simulink model "grid"  (R2014b)
settings: Solver=ode45  StartTime=0.0  StopTime=0.5  RelTol=1e-3
undefined symbols (not defined in the file): D1, Delta
libraries: powerlib x104, simulink x30
(part 1 of 2)
settings Model: Creator=quad  LastModifiedBy=SELVA
settings DataIOCC: SignalLoggingSaveFormat=ModelDataLogs
settings OptimizationCC: ExpressionDepthLimit=2147483647
settings DebuggingCC: UnderspecifiedInitializationDetection=Classic  MergeDetectMultiDrivingBlocksExec=none  FcnCallInpInsideContextMsg=UseLocalSettings  StateNameClashWarn=warning
settings GRTTargetCC: CombineOutputUpdateFcns=off  GRTInterface=on

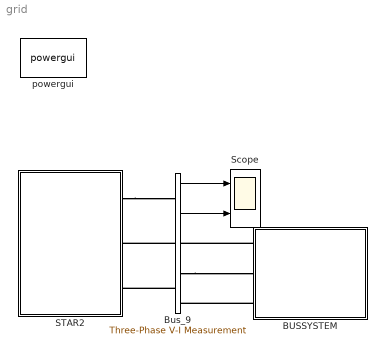
== system grid ==
  BUSSYSTEM : Subsystem
  Bus_9 : powerlib/Measurements/Three-Phase V-I Measurement  VoltageMeasurement=phase-to-phase  SetLabelV=off  LabelV=Vabc_12  Vpu=off  VpuLL=off  CurrentMeasurement=yes  SetLabelI=off  LabelI=Iabc_12  Ipu=off  Pbase=100e6  Vbase=120e3  OutputType=Complex  PhasorSimulation=on  PSBequivalent=0
  STAR2 : Subsystem
  Scope : Scope  NumInputPorts=2
      settings: YMin=-800~-3000  YMax=800~3000
  powergui : powerlib/powergui  Priority=1  SimulationMode=Discrete  SolverType=Tustin/Backward Euler (TBE)  SampleTime=5e-6  frequency=60  SPID=off  DisableSnubberDevices=off  DisableRonSwitches=off  DisableVfSwitches=off  SwTol=0  DisplayEquations=off  Interpol=off  methode=off  Ts=100  frequencyindice=50  Pbase=100e6  ErrMax=1e-4  Iterations=50  UnitsV=kV  UnitsW=MW  FunctionMessages=off  echomessages=off  HookPort=off  EnableUseOfTLC=off  x0status=blocks  RestoreLinks=warning  ResistiveCurrentMeasurement=off  Frange=[0:2:500]  Ylog=off  Xlog=on  ShowGrid=off  save=off  variable=ZData  structure=bn  ZoomFFT=off  StartTime=0.0  cycles=1  DisplayStyle=1  fundamental=60  FreqAxis=off  MaxFrequency=1000  frequencyindicesteady=1  RmsSteady=1  display=off
  wires:
  Bus_9/2 -> Scope/2
  Bus_9/1 -> Scope/1
  connections:
  STAR2/RConn1 -- Bus_9/LConn1
  Bus_9/LConn2 -- STAR2/RConn2
  Bus_9/LConn3 -- STAR2/RConn3
  BUSSYSTEM/LConn1 -- Bus_9/RConn1
  Bus_9/RConn2 -- BUSSYSTEM/LConn2
  BUSSYSTEM/LConn3 -- Bus_9/RConn3

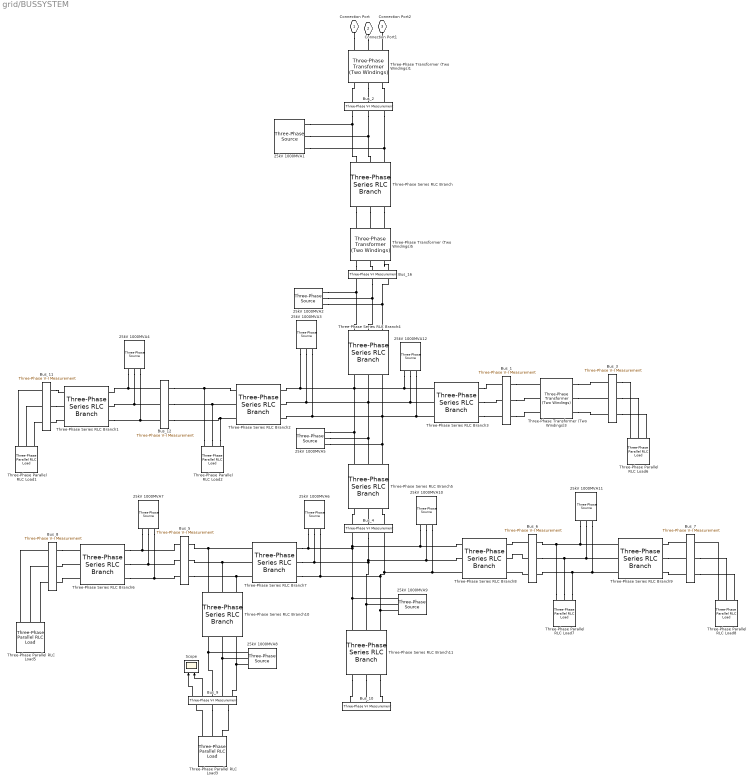
== system grid/BUSSYSTEM ==
  25kV 1000MVA{1..4,6..12} (11 alike) : powerlib/Electrical Sources/Three-Phase Source  Voltage=10  PhaseAngle=0  Frequency=50  InternalConnection=Yg  SpecifyImpedance=on  Resistance=25^2/1000/10  Inductance=25^2/1000/377  ShortCircuitLevel=1000e6  BaseVoltage=25e3  XRratio=10  BusType=swing  Pref=0  Qref=0  Qmin=-inf  Qmax=inf
  25kV 1000MVA5 : powerlib/Electrical Sources/Three-Phase Source  Voltage=25e3  PhaseAngle=0  Frequency=50  InternalConnection=Yg  SpecifyImpedance=on  Resistance=25^2/1000/10  Inductance=25^2/1000/377  ShortCircuitLevel=1000e6  BaseVoltage=25e3  XRratio=10  BusType=swing  Pref=0  Qref=0  Qmin=-inf  Qmax=inf
  Bus_1 : powerlib/Measurements/Three-Phase V-I Measurement  VoltageMeasurement=phase-to-phase  SetLabelV=on  LabelV=Vabc_5  Vpu=off  VpuLL=off  CurrentMeasurement=yes  SetLabelI=on  LabelI=Iabc_5  Ipu=off  Pbase=100e6  Vbase=120e3  OutputType=Complex  PhasorSimulation=on  PSBequivalent=0
  Bus_10 : powerlib/Measurements/Three-Phase V-I Measurement  VoltageMeasurement=phase-to-phase  SetLabelV=on  LabelV=Vabc_13  Vpu=off  VpuLL=off  CurrentMeasurement=yes  SetLabelI=on  LabelI=Iabc_13  Ipu=off  Pbase=100e6  Vbase=120e3  OutputType=Complex  PhasorSimulation=on  PSBequivalent=0
  Bus_11 : powerlib/Measurements/Three-Phase V-I Measurement  VoltageMeasurement=phase-to-phase  SetLabelV=on  LabelV=Vabc_3  Vpu=off  VpuLL=off  CurrentMeasurement=yes  SetLabelI=on  LabelI=Iabc_3  Ipu=off  Pbase=100e6  Vbase=120e3  OutputType=Complex  PhasorSimulation=on  PSBequivalent=0
  Bus_12 : powerlib/Measurements/Three-Phase V-I Measurement  VoltageMeasurement=phase-to-phase  SetLabelV=on  LabelV=Vabc_4  Vpu=off  VpuLL=off  CurrentMeasurement=yes  SetLabelI=on  LabelI=Iabc_4  Ipu=off  Pbase=100e6  Vbase=120e3  OutputType=Complex  PhasorSimulation=on  PSBequivalent=0
  Bus_16 : powerlib/Measurements/Three-Phase V-I Measurement  VoltageMeasurement=phase-to-phase  SetLabelV=on  LabelV=Vabc_1  Vpu=off  VpuLL=off  CurrentMeasurement=yes  SetLabelI=on  LabelI=Iabc_1  Ipu=off  Pbase=100e6  Vbase=120e3  OutputType=Complex  PhasorSimulation=on  PSBequivalent=0
  Bus_2 : powerlib/Measurements/Three-Phase V-I Measurement  VoltageMeasurement=phase-to-phase  SetLabelV=on  LabelV=Vabc_2  Vpu=off  VpuLL=off  CurrentMeasurement=yes  SetLabelI=on  LabelI=Iabc_2  Ipu=off  Pbase=100e6  Vbase=120e3  OutputType=Complex  PhasorSimulation=on  PSBequivalent=0
  Bus_3 : powerlib/Measurements/Three-Phase V-I Measurement  VoltageMeasurement=phase-to-phase  SetLabelV=on  LabelV=Vabc_6  Vpu=off  VpuLL=off  CurrentMeasurement=yes  SetLabelI=on  LabelI=Iabc_6  Ipu=off  Pbase=100e6  Vbase=120e3  OutputType=Complex  PhasorSimulation=on  PSBequivalent=0
  Bus_4 : powerlib/Measurements/Three-Phase V-I Measurement  VoltageMeasurement=phase-to-phase  SetLabelV=on  LabelV=Vabc_7  Vpu=off  VpuLL=off  CurrentMeasurement=yes  SetLabelI=on  LabelI=Iabc_7  Ipu=off  Pbase=100e6  Vbase=120e3  OutputType=Complex  PhasorSimulation=on  PSBequivalent=0
  Bus_5 : powerlib/Measurements/Three-Phase V-I Measurement  VoltageMeasurement=phase-to-phase  SetLabelV=on  LabelV=Vabc_8  Vpu=off  VpuLL=off  CurrentMeasurement=yes  SetLabelI=on  LabelI=Iabc_8  Ipu=off  Pbase=100e6  Vbase=120e3  OutputType=Complex  PhasorSimulation=on  PSBequivalent=0
  Bus_6 : powerlib/Measurements/Three-Phase V-I Measurement  VoltageMeasurement=phase-to-phase  SetLabelV=on  LabelV=Vabc_10  Vpu=off  VpuLL=off  CurrentMeasurement=yes  SetLabelI=on  LabelI=Iabc_10  Ipu=off  Pbase=100e6  Vbase=120e3  OutputType=Complex  PhasorSimulation=on  PSBequivalent=0
  Bus_7 : powerlib/Measurements/Three-Phase V-I Measurement  VoltageMeasurement=phase-to-phase  SetLabelV=on  LabelV=Vabc_11  Vpu=off  VpuLL=off  CurrentMeasurement=yes  SetLabelI=on  LabelI=Iabc_11  Ipu=off  Pbase=100e6  Vbase=120e3  OutputType=Complex  PhasorSimulation=on  PSBequivalent=0
  Bus_8 : powerlib/Measurements/Three-Phase V-I Measurement  VoltageMeasurement=phase-to-phase  SetLabelV=on  LabelV=Vabc_9  Vpu=off  VpuLL=off  CurrentMeasurement=yes  SetLabelI=on  LabelI=Iabc_9  Ipu=off  Pbase=100e6  Vbase=120e3  OutputType=Complex  PhasorSimulation=on  PSBequivalent=0
  Bus_9 : powerlib/Measurements/Three-Phase V-I Measurement  VoltageMeasurement=phase-to-phase  SetLabelV=off  LabelV=Vabc_12  Vpu=off  VpuLL=off  CurrentMeasurement=yes  SetLabelI=off  LabelI=Iabc_12  Ipu=off  Pbase=100e6  Vbase=120e3  OutputType=Complex  PhasorSimulation=on  PSBequivalent=0
  Scope : Scope  NumInputPorts=2
      settings: YMin=-15~-0.5  YMax=15~0.5  SaveName=ScopeData4
  Three-Phase Parallel RLC Load{1..3,5..8} (7 alike) : powerlib/Elements/Three-Phase Parallel RLC Load  LConnTagsString=A|B|C  Configuration=Y (grounded)  NominalVoltage=415  NominalFrequency=50  ActivePower=10e3  InductivePower=0  CapacitivePower=0  Measurements=None  LoadType=constant Z
  Three-Phase Series RLC Branch{,1..11} (12 alike) : powerlib/Elements/Three-Phase Series RLC Branch  LConnTagsString=A|B|C  RConnTagsString=A|B|C  BranchType=RL  Resistance=10  Inductance=1e-3  Capacitance=1e-6  Measurements=None
  Three-Phase Transformer (Two Windings)1 : powerlib/Elements/Three-Phase Transformer (Two Windings)  Winding1Connection=Delta (D1)  UNITS=pu  NominalPower=[ 1 , 50 ]  Winding1=[1.06 0.002 0.08]  Winding2Connection=Yg  Winding2=[100 0.002 0.080001]  SetSaturation=off  Rm=500  Lm=500  Saturation=[0 0;0.0023999 1.2;1 1.52]  Hysteresis=off  DataFile='hysteresis'  SetInitialFlux=off  InitialFluxes=[0.79999 -0.79999 0.70001]  Measurements=None  MoreParameters=off  BreakLoop=off  DataType=off  TransfoNumber=1
  Three-Phase Transformer (Two Windings)3 : powerlib/Elements/Three-Phase Transformer (Two Windings)  Winding1Connection=Delta (D1)  UNITS=pu  NominalPower=[ 1 , 50 ]  Winding1=[ 1.06 , 0.002 , 0.08 ]  Winding2Connection=Yg  Winding2=[ 1.06 , 0.002 , 0.08 ]  SetSaturation=off  Rm=500  Lm=500  Saturation=[ 0,0 ; 0.0024,1.2 ; 1.0,1.52 ]  Hysteresis=off  DataFile='hysteresis'  SetInitialFlux=off  InitialFluxes=[ 0.8 , -0.8 , 0.7 ]  Measurements=None  MoreParameters=off  BreakLoop=off  DataType=off  TransfoNumber=1
  Three-Phase Transformer (Two Windings)5 : powerlib/Elements/Three-Phase Transformer (Two Windings)  Winding1Connection=Delta (D1)  UNITS=pu  NominalPower=[ 1 , 50 ]  Winding1=[ 1.06 , 0.002 , 0.08 ]  Winding2Connection=Yg  Winding2=[1000 , 0.002 , 0.08 ]  SetSaturation=off  Rm=500  Lm=500  Saturation=[ 0,0 ; 0.0024,1.2 ; 1.0,1.52 ]  Hysteresis=off  DataFile='hysteresis'  SetInitialFlux=off  InitialFluxes=[ 0.8 , -0.8 , 0.7 ]  Measurements=None  MoreParameters=off  BreakLoop=off  DataType=off  TransfoNumber=1
  Connection Port : PMIOPort  Tag=PMCPort  Port=1  Side=Left
  Connection Port1 : PMIOPort  Tag=PMCPort  Port=2  Side=Left
  Connection Port2 : PMIOPort  Tag=PMCPort  Port=3  Side=Left
  wires:
  Bus_9/1 -> Scope/1
  Bus_9/2 -> Scope/2
  connections:
  Three-Phase Parallel RLC Load2/LConn3 -- Bus_12/RConn3 -- Three-Phase Series RLC Branch2/LConn3
  Three-Phase Parallel RLC Load2/LConn2 -- Three-Phase Series RLC Branch2/LConn2 -- Bus_12/RConn2
  Three-Phase Parallel RLC Load2/LConn1 -- Bus_12/RConn1 -- Three-Phase Series RLC Branch2/LConn1
  Three-Phase Series RLC Branch10/RConn2 -- Bus_5/RConn2 -- Three-Phase Series RLC Branch7/LConn2
  Three-Phase Series RLC Branch10/RConn3 -- Bus_5/RConn3 -- Three-Phase Series RLC Branch7/LConn3
  Three-Phase Series RLC Branch10/RConn1 -- Bus_5/RConn1 -- Three-Phase Series RLC Branch7/LConn1
  25kV 1000MVA12/RConn1 -- Three-Phase Series RLC Branch4/RConn1 -- Three-Phase Series RLC Branch2/RConn1 -- 25kV 1000MVA3/RConn1 -- Three-Phase Series RLC Branch5/LConn1 -- 25kV 1000MVA5/RConn1 -- Three-Phase Series RLC Branch3/LConn1
  25kV 1000MVA12/RConn2 -- Three-Phase Series RLC Branch2/RConn2 -- 25kV 1000MVA3/RConn2 -- Three-Phase Series RLC Branch4/RConn2 -- Three-Phase Series RLC Branch5/LConn2 -- 25kV 1000MVA5/RConn2 -- Three-Phase Series RLC Branch3/LConn2
  25kV 1000MVA12/RConn3 -- Three-Phase Series RLC Branch4/RConn3 -- Three-Phase Series RLC Branch2/RConn3 -- 25kV 1000MVA3/RConn3 -- Three-Phase Series RLC Branch5/LConn3 -- 25kV 1000MVA5/RConn3 -- Three-Phase Series RLC Branch3/LConn3
  25kV 1000MVA10/RConn1 -- Three-Phase Series RLC Branch7/RConn1 -- 25kV 1000MVA6/RConn1 -- Three-Phase Series RLC Branch11/LConn1 -- 25kV 1000MVA9/RConn1 -- Bus_4/LConn1 -- Three-Phase Series RLC Branch8/LConn1
  25kV 1000MVA10/RConn2 -- Three-Phase Series RLC Branch7/RConn2 -- 25kV 1000MVA6/RConn2 -- Three-Phase Series RLC Branch11/LConn2 -- 25kV 1000MVA9/RConn2 -- Bus_4/LConn2 -- Three-Phase Series RLC Branch8/LConn2
  25kV 1000MVA10/RConn3 -- Bus_4/LConn3 -- Three-Phase Series RLC Branch7/RConn3 -- 25kV 1000MVA6/RConn3 -- Three-Phase Series RLC Branch11/LConn3 -- 25kV 1000MVA9/RConn3 -- Three-Phase Series RLC Branch8/LConn3
  25kV 1000MVA4/RConn3 -- Three-Phase Series RLC Branch1/RConn3 -- Bus_12/LConn3
  25kV 1000MVA1/RConn3 -- Bus_2/LConn3 -- Three-Phase Series RLC Branch/LConn3
  25kV 1000MVA8/RConn3 -- Bus_9/RConn3 -- Three-Phase Series RLC Branch10/LConn3
  Three-Phase Parallel RLC Load7/LConn1 -- Bus_6/RConn1 -- Three-Phase Series RLC Branch9/LConn1 -- 25kV 1000MVA11/RConn1
  25kV 1000MVA4/RConn1 -- Three-Phase Series RLC Branch1/RConn1 -- Bus_12/LConn1
  25kV 1000MVA2/RConn2 -- Bus_16/LConn2 -- Three-Phase Series RLC Branch4/LConn2
  25kV 1000MVA2/RConn3 -- Bus_16/LConn3 -- Three-Phase Series RLC Branch4/LConn3
  25kV 1000MVA8/RConn1 -- Bus_9/RConn1 -- Three-Phase Series RLC Branch10/LConn1
  25kV 1000MVA2/RConn1 -- Bus_16/LConn1 -- Three-Phase Series RLC Branch4/LConn1
  25kV 1000MVA4/RConn2 -- Three-Phase Series RLC Branch1/RConn2 -- Bus_12/LConn2
  25kV 1000MVA7/RConn1 -- Three-Phase Series RLC Branch6/RConn1 -- Bus_5/LConn1
  Three-Phase Parallel RLC Load7/LConn2 -- Bus_6/RConn2 -- Three-Phase Series RLC Branch9/LConn2 -- 25kV 1000MVA11/RConn2
  25kV 1000MVA8/RConn2 -- Bus_9/RConn2 -- Three-Phase Series RLC Branch10/LConn2
  25kV 1000MVA1/RConn2 -- Bus_2/LConn2 -- Three-Phase Series RLC Branch/LConn2
  25kV 1000MVA1/RConn1 -- Bus_2/LConn1 -- Three-Phase Series RLC Branch/LConn1
  25kV 1000MVA7/RConn2 -- Three-Phase Series RLC Branch6/RConn2 -- Bus_5/LConn2
  25kV 1000MVA7/RConn3 -- Three-Phase Series RLC Branch6/RConn3 -- Bus_5/LConn3
  Three-Phase Parallel RLC Load7/LConn3 -- Bus_6/RConn3 -- Three-Phase Series RLC Branch9/LConn3 -- 25kV 1000MVA11/RConn3
  Three-Phase Series RLC Branch/RConn1 -- Three-Phase Transformer (Two Windings)5/LConn1
  Bus_7/RConn2 -- Three-Phase Parallel RLC Load8/LConn2
  Three-Phase Parallel RLC Load1/LConn2 -- Bus_11/LConn2
  Three-Phase Series RLC Branch5/RConn3 -- Bus_4/RConn3
  Three-Phase Transformer (Two Windings)3/LConn3 -- Bus_3/LConn3
  Bus_6/LConn2 -- Three-Phase Series RLC Branch8/RConn2
  Bus_1/RConn2 -- Three-Phase Transformer (Two Windings)3/RConn2
  Bus_11/RConn3 -- Three-Phase Series RLC Branch1/LConn3
  Bus_6/LConn3 -- Three-Phase Series RLC Branch8/RConn3
  Bus_8/RConn2 -- Three-Phase Series RLC Branch6/LConn2
  Three-Phase Parallel RLC Load5/LConn2 -- Bus_8/LConn2
  Three-Phase Series RLC Branch/RConn3 -- Three-Phase Transformer (Two Windings)5/LConn3
  Bus_7/RConn3 -- Three-Phase Parallel RLC Load8/LConn3
  Bus_3/RConn1 -- Three-Phase Parallel RLC Load6/LConn1
  Three-Phase Parallel RLC Load8/LConn1 -- Bus_7/RConn1
  Three-Phase Parallel RLC Load5/LConn1 -- Bus_8/LConn1
  Three-Phase Series RLC Branch11/RConn1 -- Bus_10/RConn1
  Three-Phase Transformer (Two Windings)1/RConn3 -- Bus_2/RConn3
  Three-Phase Series RLC Branch9/RConn2 -- Bus_7/LConn2
  Bus_11/RConn2 -- Three-Phase Series RLC Branch1/LConn2
  Three-Phase Series RLC Branch3/RConn3 -- Bus_1/LConn3
  Bus_9/LConn2 -- Three-Phase Parallel RLC Load3/LConn2
  Three-Phase Transformer (Two Windings)3/LConn1 -- Bus_3/LConn1
  Three-Phase Series RLC Branch3/RConn1 -- Bus_1/LConn1
  Three-Phase Parallel RLC Load5/LConn3 -- Bus_8/LConn3
  Three-Phase Parallel RLC Load1/LConn3 -- Bus_11/LConn3
  Three-Phase Transformer (Two Windings)5/RConn2 -- Bus_16/RConn2
  Three-Phase Series RLC Branch3/RConn2 -- Bus_1/LConn2
  Three-Phase Series RLC Branch9/RConn3 -- Bus_7/LConn3
  Bus_9/LConn3 -- Three-Phase Parallel RLC Load3/LConn3
  Bus_6/LConn1 -- Three-Phase Series RLC Branch8/RConn1
  Bus_1/RConn3 -- Three-Phase Transformer (Two Windings)3/RConn3
  Bus_4/RConn2 -- Three-Phase Series RLC Branch5/RConn2
  Bus_3/RConn3 -- Three-Phase Parallel RLC Load6/LConn3
  Bus_8/RConn3 -- Three-Phase Series RLC Branch6/LConn3
  Three-Phase Series RLC Branch11/RConn2 -- Bus_10/RConn2
  Bus_1/RConn1 -- Three-Phase Transformer (Two Windings)3/RConn1
  Three-Phase Series RLC Branch11/RConn3 -- Bus_10/RConn3
  Three-Phase Transformer (Two Windings)3/LConn2 -- Bus_3/LConn2
  Three-Phase Transformer (Two Windings)1/RConn2 -- Bus_2/RConn2
  Bus_3/RConn2 -- Three-Phase Parallel RLC Load6/LConn2
  Three-Phase Transformer (Two Windings)5/RConn1 -- Bus_16/RConn1
  Three-Phase Series RLC Branch9/RConn1 -- Bus_7/LConn1
  Three-Phase Parallel RLC Load3/LConn1 -- Bus_9/LConn1
  Bus_11/RConn1 -- Three-Phase Series RLC Branch1/LConn1
  Three-Phase Parallel RLC Load1/LConn1 -- Bus_11/LConn1
  Bus_4/RConn1 -- Three-Phase Series RLC Branch5/RConn1
  Three-Phase Transformer (Two Windings)1/RConn1 -- Bus_2/RConn1
  Three-Phase Series RLC Branch/RConn2 -- Three-Phase Transformer (Two Windings)5/LConn2
  Three-Phase Transformer (Two Windings)5/RConn3 -- Bus_16/RConn3
  Connection Port1/RConn1 -- Three-Phase Transformer (Two Windings)1/LConn2
  Bus_8/RConn1 -- Three-Phase Series RLC Branch6/LConn1
  Connection Port/RConn1 -- Three-Phase Transformer (Two Windings)1/LConn1
  Connection Port2/RConn1 -- Three-Phase Transformer (Two Windings)1/LConn3

== system grid/STAR2 ==
  "B " : Subsystem
  DC : Subsystem
  DC1 : Subsystem
  DC2 : Subsystem
  Ground : powerlib/Elements/Ground  LConnTagsString=a
  R : Subsystem
  Y : Subsystem
  A : PMIOPort  Tag=PMCPort  Port=1  Side=Right
  B : PMIOPort  Tag=PMCPort  Port=2  Side=Right
  C : PMIOPort  Tag=PMCPort  Port=3  Side=Right
  connections:
  R/RConn2 -- Y/RConn2 -- "B "/RConn2 -- Ground/LConn1
  DC/RConn1 -- R/LConn1
  DC/RConn3 -- R/LConn3
  DC/RConn4 -- R/LConn4
  DC/RConn9 -- R/LConn9
  DC/RConn2 -- R/LConn2
  DC/RConn5 -- R/LConn5
  DC/RConn7 -- R/LConn7
  DC/RConn6 -- R/LConn6
  DC/RConn8 -- R/LConn8
  DC/RConn10 -- R/LConn10
  DC1/RConn1 -- Y/LConn1
  DC1/RConn2 -- Y/LConn2
  DC1/RConn3 -- Y/LConn3
  DC1/RConn4 -- Y/LConn4
  DC1/RConn5 -- Y/LConn5
  DC1/RConn6 -- Y/LConn6
  DC1/RConn7 -- Y/LConn7
  DC1/RConn8 -- Y/LConn8
  DC1/RConn9 -- Y/LConn9
  DC1/RConn10 -- Y/LConn10
  DC2/RConn1 -- "B "/LConn1
  DC2/RConn2 -- "B "/LConn2
  DC2/RConn3 -- "B "/LConn3
  DC2/RConn4 -- "B "/LConn4
  DC2/RConn5 -- "B "/LConn5
  DC2/RConn6 -- "B "/LConn6
  DC2/RConn7 -- "B "/LConn7
  DC2/RConn8 -- "B "/LConn8
  DC2/RConn9 -- "B "/LConn9
  DC2/RConn10 -- "B "/LConn10
  Y/RConn1 -- B/RConn1
  R/RConn1 -- A/RConn1
  "B "/RConn1 -- C/RConn1

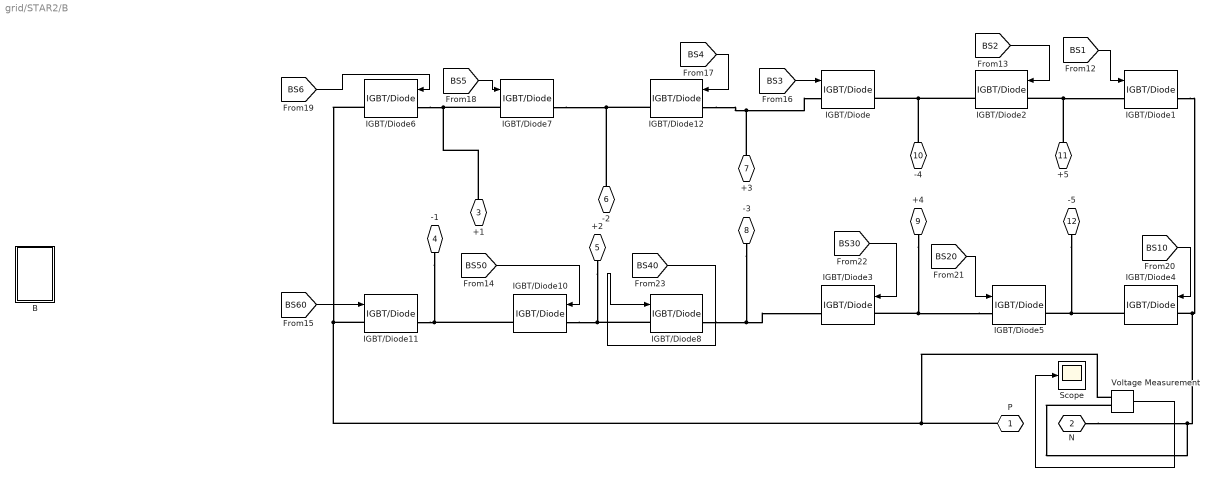
== system grid/STAR2/B  ==
  B : Subsystem  mask{fc=1000, m=1}
      mask prompts: fc "Switching frequency"; m "modulation index"
  IGBT/Diode{,1..8,10..12} (12 alike) : powerlib/Power Electronics/IGBT//Diode  Ron=1e-3  Rs=1e5  Cs=inf  Measurements=on
  Scope : Scope
  Voltage Measurement : powerlib/Measurements/Voltage Measurement  PhasorSimulation=off  OutputType=Complex  PSBequivalent=0
  P : PMIOPort  Tag=PMCPort  Port=1  Side=Right
  N : PMIOPort  Tag=PMCPort  Port=2  Side=Right
  +1 : PMIOPort  Tag=PMCPort  Port=3  Side=Left
  -1 : PMIOPort  Tag=PMCPort  Port=4  Side=Left
  +2 : PMIOPort  Tag=PMCPort  Port=5  Side=Left
  -2 : PMIOPort  Tag=PMCPort  Port=6  Side=Left
  +3 : PMIOPort  Tag=PMCPort  Port=7  Side=Left
  -3 : PMIOPort  Tag=PMCPort  Port=8  Side=Left
  +4 : PMIOPort  Tag=PMCPort  Port=9  Side=Left
  -4 : PMIOPort  Tag=PMCPort  Port=10  Side=Left
  +5 : PMIOPort  Tag=PMCPort  Port=11  Side=Left
  -5 : PMIOPort  Tag=PMCPort  Port=12  Side=Left
  wires:
  [BS10] -> IGBT/Diode4/1
  [BS2] -> IGBT/Diode2/1
  [BS20] -> IGBT/Diode5/1
  [BS3] -> IGBT/Diode/1
  [BS30] -> IGBT/Diode3/1
  [BS40] -> IGBT/Diode8/1
  [BS6] -> IGBT/Diode6/1
  [BS4] -> IGBT/Diode12/1
  [BS5] -> IGBT/Diode7/1
  [BS50] -> IGBT/Diode10/1
  [BS60] -> IGBT/Diode11/1
  Voltage Measurement/1 -> Scope/1
  [BS1] -> IGBT/Diode1/1
  connections:
  IGBT/Diode2/RConn1 -- -4/RConn1 -- IGBT/Diode/RConn1
  IGBT/Diode2/LConn1 -- IGBT/Diode1/LConn1 -- +5/RConn1
  IGBT/Diode5/LConn1 -- +4/RConn1 -- IGBT/Diode3/LConn1
  IGBT/Diode4/RConn1 -- -5/RConn1 -- IGBT/Diode5/RConn1
  IGBT/Diode4/LConn1 -- IGBT/Diode1/RConn1 -- N/RConn1 -- Voltage Measurement/LConn2
  IGBT/Diode7/LConn1 -- +1/RConn1 -- IGBT/Diode6/LConn1
  IGBT/Diode12/RConn1 -- IGBT/Diode7/RConn1 -- -2/RConn1
  IGBT/Diode10/RConn1 -- IGBT/Diode11/RConn1 -- -1/RConn1
  IGBT/Diode8/LConn1 -- IGBT/Diode10/LConn1 -- +2/RConn1
  IGBT/Diode12/LConn1 -- IGBT/Diode/LConn1 -- +3/RConn1
  IGBT/Diode8/RConn1 -- IGBT/Diode3/RConn1 -- -3/RConn1
  IGBT/Diode6/RConn1 -- IGBT/Diode11/LConn1 -- P/RConn1 -- Voltage Measurement/LConn1

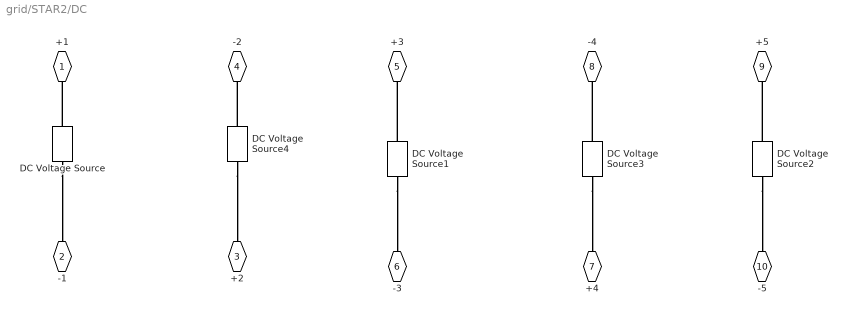
== system grid/STAR2/DC ==
  DC Voltage Source{,1..4} (5 alike) : powerlib/Electrical Sources/DC Voltage Source  Amplitude=66.5  Measurements=None
  +1 : PMIOPort  Tag=PMCPort  Port=1  Side=Right
  -1 : PMIOPort  Tag=PMCPort  Port=2  Side=Right
  +2 : PMIOPort  Tag=PMCPort  Port=3  Side=Right
  -2 : PMIOPort  Tag=PMCPort  Port=4  Side=Right
  +3 : PMIOPort  Tag=PMCPort  Port=5  Side=Right
  -3 : PMIOPort  Tag=PMCPort  Port=6  Side=Right
  +4 : PMIOPort  Tag=PMCPort  Port=7  Side=Right
  -4 : PMIOPort  Tag=PMCPort  Port=8  Side=Right
  +5 : PMIOPort  Tag=PMCPort  Port=9  Side=Right
  -5 : PMIOPort  Tag=PMCPort  Port=10  Side=Right
  connections:
  DC Voltage Source/LConn1 -- -1/RConn1
  DC Voltage Source/RConn1 -- +1/RConn1
  DC Voltage Source1/LConn1 -- -3/RConn1
  DC Voltage Source3/RConn1 -- +4/RConn1
  DC Voltage Source2/LConn1 -- -5/RConn1
  DC Voltage Source1/RConn1 -- +3/RConn1
  DC Voltage Source2/RConn1 -- +5/RConn1
  DC Voltage Source3/LConn1 -- -4/RConn1
  DC Voltage Source4/LConn1 -- -2/RConn1
  DC Voltage Source4/RConn1 -- +2/RConn1

== system grid/STAR2/DC1 ==
  DC Voltage Source{,1..4} (5 alike) : powerlib/Electrical Sources/DC Voltage Source  Amplitude=66.5  Measurements=None
  +1 : PMIOPort  Tag=PMCPort  Port=1  Side=Right
  -1 : PMIOPort  Tag=PMCPort  Port=2  Side=Right
  +2 : PMIOPort  Tag=PMCPort  Port=3  Side=Right
  -2 : PMIOPort  Tag=PMCPort  Port=4  Side=Right
  +3 : PMIOPort  Tag=PMCPort  Port=5  Side=Right
  -3 : PMIOPort  Tag=PMCPort  Port=6  Side=Right
  +4 : PMIOPort  Tag=PMCPort  Port=7  Side=Right
  -4 : PMIOPort  Tag=PMCPort  Port=8  Side=Right
  +5 : PMIOPort  Tag=PMCPort  Port=9  Side=Right
  -5 : PMIOPort  Tag=PMCPort  Port=10  Side=Right
  connections:
  DC Voltage Source4/RConn1 -- +2/RConn1
  DC Voltage Source4/LConn1 -- -2/RConn1
  DC Voltage Source3/LConn1 -- -4/RConn1
  DC Voltage Source2/RConn1 -- +5/RConn1
  DC Voltage Source1/RConn1 -- +3/RConn1
  DC Voltage Source2/LConn1 -- -5/RConn1
  DC Voltage Source3/RConn1 -- +4/RConn1
  DC Voltage Source1/LConn1 -- -3/RConn1
  DC Voltage Source/RConn1 -- +1/RConn1
  DC Voltage Source/LConn1 -- -1/RConn1

== system grid/STAR2/DC2 ==
  DC Voltage Source{,1..4} (5 alike) : powerlib/Electrical Sources/DC Voltage Source  Amplitude=66.5  Measurements=None
  +1 : PMIOPort  Tag=PMCPort  Port=1  Side=Right
  -1 : PMIOPort  Tag=PMCPort  Port=2  Side=Right
  +2 : PMIOPort  Tag=PMCPort  Port=3  Side=Right
  -2 : PMIOPort  Tag=PMCPort  Port=4  Side=Right
  +3 : PMIOPort  Tag=PMCPort  Port=5  Side=Right
  -3 : PMIOPort  Tag=PMCPort  Port=6  Side=Right
  +4 : PMIOPort  Tag=PMCPort  Port=7  Side=Right
  -4 : PMIOPort  Tag=PMCPort  Port=8  Side=Right
  +5 : PMIOPort  Tag=PMCPort  Port=9  Side=Right
  -5 : PMIOPort  Tag=PMCPort  Port=10  Side=Right
  connections:
  DC Voltage Source/LConn1 -- -1/RConn1
  DC Voltage Source/RConn1 -- +1/RConn1
  DC Voltage Source1/LConn1 -- -3/RConn1
  DC Voltage Source3/RConn1 -- +4/RConn1
  DC Voltage Source2/LConn1 -- -5/RConn1
  DC Voltage Source1/RConn1 -- +3/RConn1
  DC Voltage Source2/RConn1 -- +5/RConn1
  DC Voltage Source3/LConn1 -- -4/RConn1
  DC Voltage Source4/LConn1 -- -2/RConn1
  DC Voltage Source4/RConn1 -- +2/RConn1

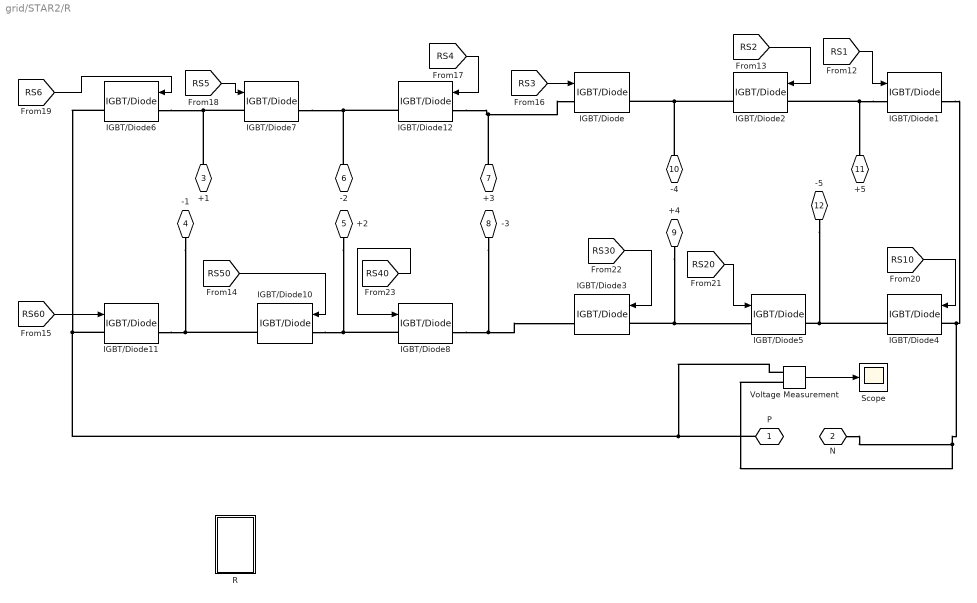
== system grid/STAR2/R ==
  IGBT/Diode{,1..8,10..12} (12 alike) : powerlib/Power Electronics/IGBT//Diode  Ron=1e-3  Rs=1e5  Cs=inf  Measurements=on
  R : Subsystem  mask{fc=1000, m=1}
      mask prompts: fc "Switching frequency"; m "modulation index"
  Scope : Scope
  Voltage Measurement : powerlib/Measurements/Voltage Measurement  PhasorSimulation=off  OutputType=Complex  PSBequivalent=0
  P : PMIOPort  Tag=PMCPort  Port=1  Side=Right
  N : PMIOPort  Tag=PMCPort  Port=2  Side=Right
  +1 : PMIOPort  Tag=PMCPort  Port=3  Side=Left
  -1 : PMIOPort  Tag=PMCPort  Port=4  Side=Left
  +2 : PMIOPort  Tag=PMCPort  Port=5  Side=Left
  -2 : PMIOPort  Tag=PMCPort  Port=6  Side=Left
  +3 : PMIOPort  Tag=PMCPort  Port=7  Side=Left
  -3 : PMIOPort  Tag=PMCPort  Port=8  Side=Left
  +4 : PMIOPort  Tag=PMCPort  Port=9  Side=Left
  -4 : PMIOPort  Tag=PMCPort  Port=10  Side=Left
  +5 : PMIOPort  Tag=PMCPort  Port=11  Side=Left
  -5 : PMIOPort  Tag=PMCPort  Port=12  Side=Left
  wires:
  [RS10] -> IGBT/Diode4/1
  [RS2] -> IGBT/Diode2/1
  [RS20] -> IGBT/Diode5/1
  [RS3] -> IGBT/Diode/1
  [RS30] -> IGBT/Diode3/1
  [RS40] -> IGBT/Diode8/1
  [RS6] -> IGBT/Diode6/1
  [RS4] -> IGBT/Diode12/1
  [RS5] -> IGBT/Diode7/1
  [RS50] -> IGBT/Diode10/1
  [RS60] -> IGBT/Diode11/1
  Voltage Measurement/1 -> Scope/1
  [RS1] -> IGBT/Diode1/1
  connections:
  IGBT/Diode2/RConn1 -- -4/RConn1 -- IGBT/Diode/RConn1
  IGBT/Diode1/LConn1 -- IGBT/Diode2/LConn1 -- +5/RConn1
  +4/RConn1 -- IGBT/Diode5/LConn1 -- IGBT/Diode3/LConn1
  IGBT/Diode4/RConn1 -- -5/RConn1 -- IGBT/Diode5/RConn1
  IGBT/Diode4/LConn1 -- Voltage Measurement/LConn2 -- N/RConn1 -- IGBT/Diode1/RConn1
  IGBT/Diode7/LConn1 -- IGBT/Diode6/LConn1 -- +1/RConn1
  IGBT/Diode12/RConn1 -- -2/RConn1 -- IGBT/Diode7/RConn1
  IGBT/Diode10/RConn1 -- IGBT/Diode11/RConn1 -- -1/RConn1
  IGBT/Diode8/LConn1 -- +2/RConn1 -- IGBT/Diode10/LConn1
  IGBT/Diode12/LConn1 -- IGBT/Diode/LConn1 -- +3/RConn1
  IGBT/Diode8/RConn1 -- IGBT/Diode3/RConn1 -- -3/RConn1
  IGBT/Diode6/RConn1 -- Voltage Measurement/LConn1 -- P/RConn1 -- IGBT/Diode11/LConn1

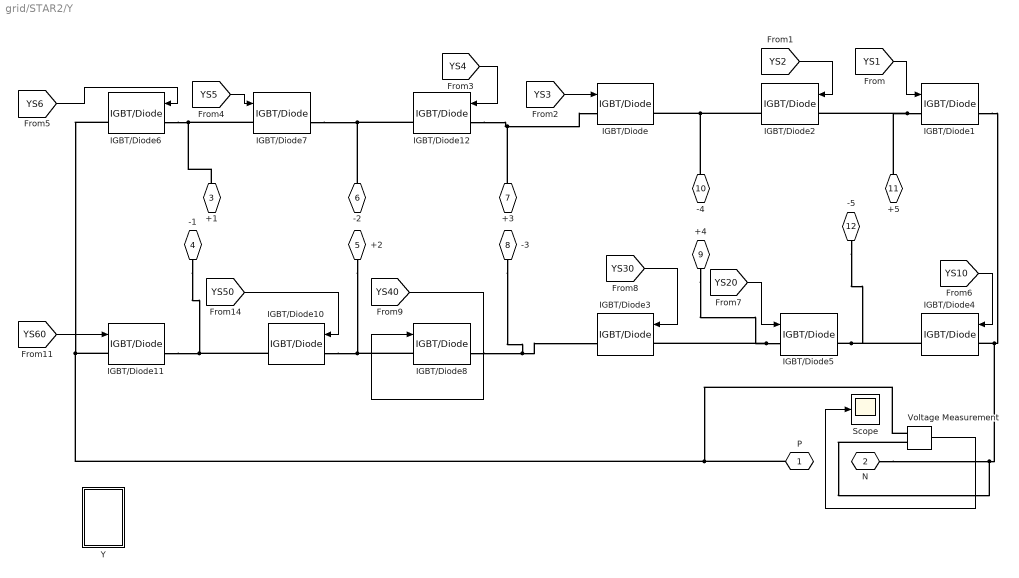
== system grid/STAR2/Y ==
  IGBT/Diode{,1..8,10..12} (12 alike) : powerlib/Power Electronics/IGBT//Diode  Ron=1e-3  Rs=1e5  Cs=inf  Measurements=on
  Scope : Scope
  Voltage Measurement : powerlib/Measurements/Voltage Measurement  PhasorSimulation=off  OutputType=Complex  PSBequivalent=0
  Y : Subsystem  mask{fc=1000, m=1}
      mask prompts: fc "Switching frequency"; m "modulation index"
  P : PMIOPort  Tag=PMCPort  Port=1  Side=Right
  N : PMIOPort  Tag=PMCPort  Port=2  Side=Right
  +1 : PMIOPort  Tag=PMCPort  Port=3  Side=Left
  -1 : PMIOPort  Tag=PMCPort  Port=4  Side=Left
  +2 : PMIOPort  Tag=PMCPort  Port=5  Side=Left
  -2 : PMIOPort  Tag=PMCPort  Port=6  Side=Left
  +3 : PMIOPort  Tag=PMCPort  Port=7  Side=Left
  -3 : PMIOPort  Tag=PMCPort  Port=8  Side=Left
  +4 : PMIOPort  Tag=PMCPort  Port=9  Side=Left
  -4 : PMIOPort  Tag=PMCPort  Port=10  Side=Left
  +5 : PMIOPort  Tag=PMCPort  Port=11  Side=Left
  -5 : PMIOPort  Tag=PMCPort  Port=12  Side=Left
  wires:
  [YS1] -> IGBT/Diode1/1
  Voltage Measurement/1 -> Scope/1
  [YS60] -> IGBT/Diode11/1
  [YS50] -> IGBT/Diode10/1
  [YS5] -> IGBT/Diode7/1
  [YS4] -> IGBT/Diode12/1
  [YS6] -> IGBT/Diode6/1
  [YS40] -> IGBT/Diode8/1
  [YS30] -> IGBT/Diode3/1
  [YS3] -> IGBT/Diode/1
  [YS20] -> IGBT/Diode5/1
  [YS2] -> IGBT/Diode2/1
  [YS10] -> IGBT/Diode4/1
  connections:
  Voltage Measurement/LConn1 -- P/RConn1 -- IGBT/Diode11/LConn1 -- IGBT/Diode6/RConn1
  IGBT/Diode8/RConn1 -- -3/RConn1 -- IGBT/Diode3/RConn1
  IGBT/Diode12/LConn1 -- +3/RConn1 -- IGBT/Diode/LConn1
  IGBT/Diode10/LConn1 -- IGBT/Diode8/LConn1 -- +2/RConn1
  IGBT/Diode11/RConn1 -- IGBT/Diode10/RConn1 -- -1/RConn1
  IGBT/Diode7/RConn1 -- IGBT/Diode12/RConn1 -- -2/RConn1
  IGBT/Diode6/LConn1 -- IGBT/Diode7/LConn1 -- +1/RConn1
  Voltage Measurement/LConn2 -- N/RConn1 -- IGBT/Diode1/RConn1 -- IGBT/Diode4/LConn1
  IGBT/Diode5/RConn1 -- IGBT/Diode4/RConn1 -- -5/RConn1
  IGBT/Diode5/LConn1 -- IGBT/Diode3/LConn1 -- +4/RConn1
  IGBT/Diode1/LConn1 -- IGBT/Diode2/LConn1 -- +5/RConn1
  IGBT/Diode2/RConn1 -- IGBT/Diode/RConn1 -- -4/RConn1

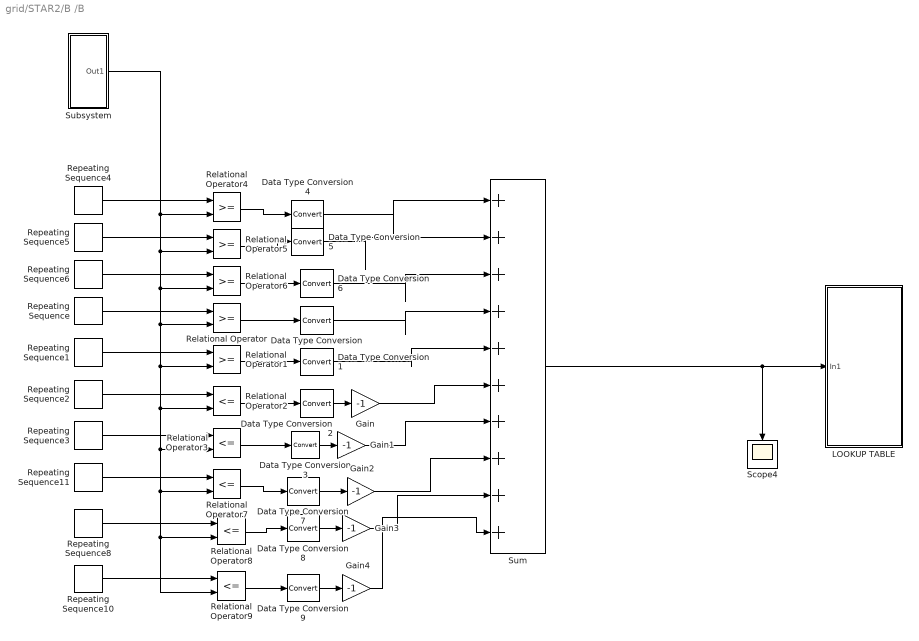
== system grid/STAR2/B /B ==
  Data Type Conversion{,1..9} (10 alike) : DataTypeConversion
  Gain{,1..4} (5 alike) : Gain  Gain=-1
  LOOKUP TABLE : Subsystem
  Relational Operator{,1,4..6} (5 alike) : RelationalOperator  OutDataTypeStr=boolean
  Relational Operator{2..3,7..9} (5 alike) : RelationalOperator  Operator=<=  OutDataTypeStr=boolean
  Repeating Sequence : simulink/Sources/Repeating Sequence  rep_seq_t="[0 (1/fc)/2  (1/fc)]"  rep_seq_y=[2 1 2]
  Repeating Sequence1 : simulink/Sources/Repeating Sequence  rep_seq_t="[0 (1/fc)/2  (1/fc)]"  rep_seq_y=[1 0 1]
  Repeating Sequence10 : simulink/Sources/Repeating Sequence  rep_seq_t="[0 (1/fc)/2  (1/fc)]"  rep_seq_y=[-5 -4 -5]
  Repeating Sequence11 : simulink/Sources/Repeating Sequence  rep_seq_t="[0 (1/fc)/2  (1/fc)]"  rep_seq_y=[-3 -2 -3]
  Repeating Sequence2 : simulink/Sources/Repeating Sequence  rep_seq_t="[0 (1/fc)/2  (1/fc)]"  rep_seq_y=[-1 0 -1]
  Repeating Sequence3 : simulink/Sources/Repeating Sequence  rep_seq_t="[0 (1/fc)/2  (1/fc)]"  rep_seq_y=[-2 -1 -2]
  Repeating Sequence4 : simulink/Sources/Repeating Sequence  rep_seq_t="[0 (1/fc)/2  (1/fc)]"  rep_seq_y=[4 5 4]
  Repeating Sequence5 : simulink/Sources/Repeating Sequence  rep_seq_t="[0 (1/fc)/2  (1/fc)]"  rep_seq_y=[4 3 4]
  Repeating Sequence6 : simulink/Sources/Repeating Sequence  rep_seq_t="[0 (1/fc)/2  (1/fc)]"  rep_seq_y=[3 2 3]
  Repeating Sequence8 : simulink/Sources/Repeating Sequence  rep_seq_t="[0 (1/fc)/2  (1/fc)]"  rep_seq_y=[-4 -3 -4]
  Scope4 : Scope
      settings: SaveName=ScopeData8
  Subsystem : Subsystem
  Sum : Sum  Inputs=|++++++++++
  wires:
  Subsystem/1(Out1) -> Relational Operator5/2, Relational Operator6/2, Relational Operator1/2, Relational Operator2/2, Relational Operator3/2, Relational Operator7/2, Relational Operator9/2, Relational Operator8/2, Relational Operator/2, Relational Operator4/2
  Sum/1 -> LOOKUP TABLE/1(In1), Scope4/1
  Gain4/1 -> Sum/10
  Gain3/1 -> Sum/9
  Gain2/1 -> Sum/8
  Gain1/1 -> Sum/7
  Gain/1 -> Sum/6
  Data Type Conversion1/1 -> Sum/5
  Data Type Conversion/1 -> Sum/4
  Data Type Conversion6/1 -> Sum/3
  Data Type Conversion5/1 -> Sum/2
  Data Type Conversion4/1 -> Sum/1
  Repeating Sequence10/1 -> Relational Operator9/1
  Data Type Conversion7/1 -> Gain2/1
  Data Type Conversion8/1 -> Gain3/1
  Data Type Conversion9/1 -> Gain4/1
  Relational Operator7/1 -> Data Type Conversion7/1
  Relational Operator8/1 -> Data Type Conversion8/1
  Relational Operator9/1 -> Data Type Conversion9/1
  Repeating Sequence11/1 -> Relational Operator7/1
  Repeating Sequence8/1 -> Relational Operator8/1
  Relational Operator4/1 -> Data Type Conversion4/1
  Relational Operator5/1 -> Data Type Conversion5/1
  Relational Operator6/1 -> Data Type Conversion6/1
  Repeating Sequence4/1 -> Relational Operator4/1
  Repeating Sequence5/1 -> Relational Operator5/1
  Repeating Sequence6/1 -> Relational Operator6/1
  Relational Operator/1 -> Data Type Conversion/1
  Relational Operator1/1 -> Data Type Conversion1/1
  Repeating Sequence/1 -> Relational Operator/1
  Repeating Sequence1/1 -> Relational Operator1/1
  Repeating Sequence2/1 -> Relational Operator2/1
  Repeating Sequence3/1 -> Relational Operator3/1
  Relational Operator2/1 -> Data Type Conversion2/1
  Relational Operator3/1 -> Data Type Conversion3/1
  Data Type Conversion2/1 -> Gain/1
  Data Type Conversion3/1 -> Gain1/1

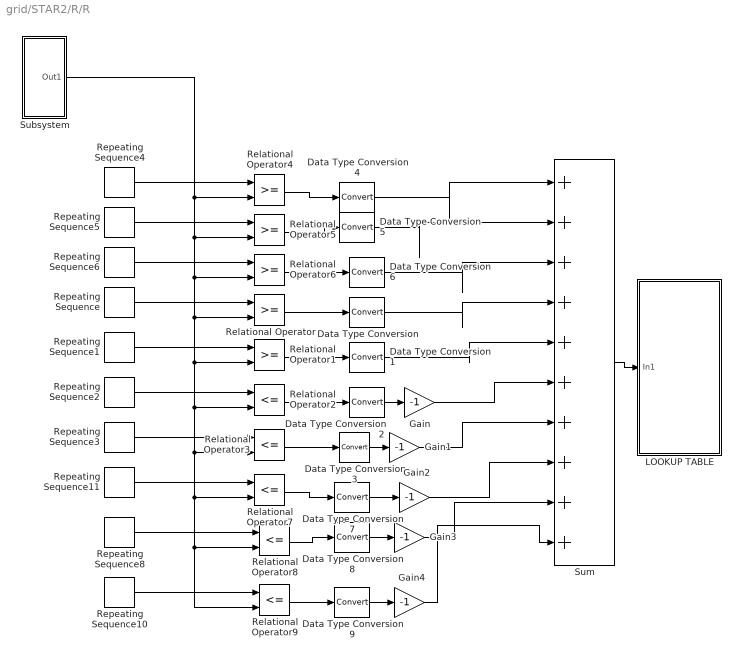
== system grid/STAR2/R/R ==
  Data Type Conversion{,1..9} (10 alike) : DataTypeConversion
  Gain{,1..4} (5 alike) : Gain  Gain=-1
  LOOKUP TABLE : Subsystem
  Relational Operator{,1,4..6} (5 alike) : RelationalOperator  OutDataTypeStr=boolean
  Relational Operator{2..3,7..9} (5 alike) : RelationalOperator  Operator=<=  OutDataTypeStr=boolean
  Repeating Sequence : simulink/Sources/Repeating Sequence  rep_seq_t="[0 (1/fc)/2  (1/fc)]"  rep_seq_y=[2 1 2]
  Repeating Sequence1 : simulink/Sources/Repeating Sequence  rep_seq_t="[0 (1/fc)/2  (1/fc)]"  rep_seq_y=[1 0 1]
  Repeating Sequence10 : simulink/Sources/Repeating Sequence  rep_seq_t="[0 (1/fc)/2  (1/fc)]"  rep_seq_y=[-5 -4 -5]
  Repeating Sequence11 : simulink/Sources/Repeating Sequence  rep_seq_t="[0 (1/fc)/2  (1/fc)]"  rep_seq_y=[-3 -2 -3]
  Repeating Sequence2 : simulink/Sources/Repeating Sequence  rep_seq_t="[0 (1/fc)/2  (1/fc)]"  rep_seq_y=[-1 0 -1]
  Repeating Sequence3 : simulink/Sources/Repeating Sequence  rep_seq_t="[0 (1/fc)/2  (1/fc)]"  rep_seq_y=[-2 -1 -2]
  Repeating Sequence4 : simulink/Sources/Repeating Sequence  rep_seq_t="[0 (1/fc)/2  (1/fc)]"  rep_seq_y=[4 5 4]
  Repeating Sequence5 : simulink/Sources/Repeating Sequence  rep_seq_t="[0 (1/fc)/2  (1/fc)]"  rep_seq_y=[4 3 4]
  Repeating Sequence6 : simulink/Sources/Repeating Sequence  rep_seq_t="[0 (1/fc)/2  (1/fc)]"  rep_seq_y=[3 2 3]
  Repeating Sequence8 : simulink/Sources/Repeating Sequence  rep_seq_t="[0 (1/fc)/2  (1/fc)]"  rep_seq_y=[-4 -3 -4]
  Subsystem : Subsystem
  Sum : Sum  Inputs=|++++++++++
  wires:
  Subsystem/1(Out1) -> Relational Operator4/2, Relational Operator5/2, Relational Operator6/2, Relational Operator7/2, Relational Operator9/2, Relational Operator8/2, Relational Operator3/2, Relational Operator2/2, Relational Operator1/2, Relational Operator/2
  Sum/1 -> LOOKUP TABLE/1(In1)
  Gain4/1 -> Sum/10
  Gain3/1 -> Sum/9
  Gain2/1 -> Sum/8
  Gain1/1 -> Sum/7
  Gain/1 -> Sum/6
  Data Type Conversion1/1 -> Sum/5
  Data Type Conversion/1 -> Sum/4
  Data Type Conversion6/1 -> Sum/3
  Data Type Conversion5/1 -> Sum/2
  Data Type Conversion4/1 -> Sum/1
  Repeating Sequence10/1 -> Relational Operator9/1
  Data Type Conversion7/1 -> Gain2/1
  Data Type Conversion8/1 -> Gain3/1
  Data Type Conversion9/1 -> Gain4/1
  Relational Operator7/1 -> Data Type Conversion7/1
  Relational Operator8/1 -> Data Type Conversion8/1
  Relational Operator9/1 -> Data Type Conversion9/1
  Repeating Sequence11/1 -> Relational Operator7/1
  Repeating Sequence8/1 -> Relational Operator8/1
  Relational Operator4/1 -> Data Type Conversion4/1
  Relational Operator5/1 -> Data Type Conversion5/1
  Relational Operator6/1 -> Data Type Conversion6/1
  Repeating Sequence4/1 -> Relational Operator4/1
  Repeating Sequence5/1 -> Relational Operator5/1
  Repeating Sequence6/1 -> Relational Operator6/1
  Relational Operator/1 -> Data Type Conversion/1
  Relational Operator1/1 -> Data Type Conversion1/1
  Repeating Sequence/1 -> Relational Operator/1
  Repeating Sequence1/1 -> Relational Operator1/1
  Repeating Sequence2/1 -> Relational Operator2/1
  Repeating Sequence3/1 -> Relational Operator3/1
  Relational Operator2/1 -> Data Type Conversion2/1
  Relational Operator3/1 -> Data Type Conversion3/1
  Data Type Conversion2/1 -> Gain/1
  Data Type Conversion3/1 -> Gain1/1

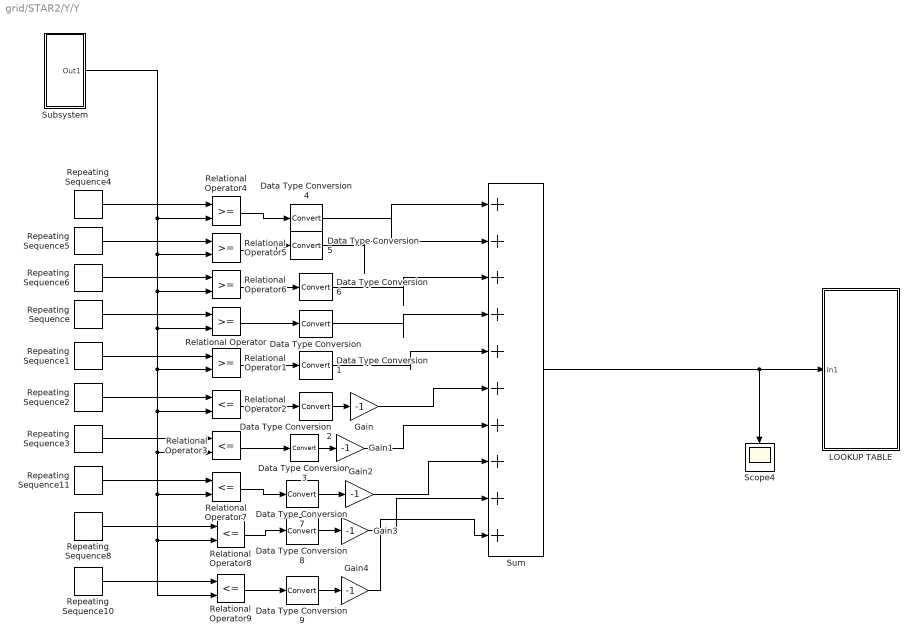
== system grid/STAR2/Y/Y ==
  Data Type Conversion{,1..9} (10 alike) : DataTypeConversion
  Gain{,1..4} (5 alike) : Gain  Gain=-1
  LOOKUP TABLE : Subsystem
  Relational Operator{,1,4..6} (5 alike) : RelationalOperator  OutDataTypeStr=boolean
  Relational Operator{2..3,7..9} (5 alike) : RelationalOperator  Operator=<=  OutDataTypeStr=boolean
  Repeating Sequence : simulink/Sources/Repeating Sequence  rep_seq_t="[0 (1/fc)/2  (1/fc)]"  rep_seq_y=[2 1 2]
  Repeating Sequence1 : simulink/Sources/Repeating Sequence  rep_seq_t="[0 (1/fc)/2  (1/fc)]"  rep_seq_y=[1 0 1]
  Repeating Sequence10 : simulink/Sources/Repeating Sequence  rep_seq_t="[0 (1/fc)/2  (1/fc)]"  rep_seq_y=[-5 -4 -5]
  Repeating Sequence11 : simulink/Sources/Repeating Sequence  rep_seq_t="[0 (1/fc)/2  (1/fc)]"  rep_seq_y=[-3 -2 -3]
  Repeating Sequence2 : simulink/Sources/Repeating Sequence  rep_seq_t="[0 (1/fc)/2  (1/fc)]"  rep_seq_y=[-1 0 -1]
  Repeating Sequence3 : simulink/Sources/Repeating Sequence  rep_seq_t="[0 (1/fc)/2  (1/fc)]"  rep_seq_y=[-2 -1 -2]
  Repeating Sequence4 : simulink/Sources/Repeating Sequence  rep_seq_t="[0 (1/fc)/2  (1/fc)]"  rep_seq_y=[4 5 4]
  Repeating Sequence5 : simulink/Sources/Repeating Sequence  rep_seq_t="[0 (1/fc)/2  (1/fc)]"  rep_seq_y=[4 3 4]
  Repeating Sequence6 : simulink/Sources/Repeating Sequence  rep_seq_t="[0 (1/fc)/2  (1/fc)]"  rep_seq_y=[3 2 3]
  Repeating Sequence8 : simulink/Sources/Repeating Sequence  rep_seq_t="[0 (1/fc)/2  (1/fc)]"  rep_seq_y=[-4 -3 -4]
  Scope4 : Scope
      settings: SaveName=ScopeData8
  Subsystem : Subsystem
  Sum : Sum  Inputs=|++++++++++
  wires:
  Subsystem/1(Out1) -> Relational Operator4/2, Relational Operator/2, Relational Operator9/2, Relational Operator8/2, Relational Operator7/2, Relational Operator3/2, Relational Operator2/2, Relational Operator1/2, Relational Operator6/2, Relational Operator5/2
  Data Type Conversion3/1 -> Gain1/1
  Data Type Conversion2/1 -> Gain/1
  Relational Operator3/1 -> Data Type Conversion3/1
  Relational Operator2/1 -> Data Type Conversion2/1
  Repeating Sequence3/1 -> Relational Operator3/1
  Repeating Sequence2/1 -> Relational Operator2/1
  Repeating Sequence1/1 -> Relational Operator1/1
  Repeating Sequence/1 -> Relational Operator/1
  Relational Operator1/1 -> Data Type Conversion1/1
  Relational Operator/1 -> Data Type Conversion/1
  Repeating Sequence6/1 -> Relational Operator6/1
  Repeating Sequence5/1 -> Relational Operator5/1
  Repeating Sequence4/1 -> Relational Operator4/1
  Relational Operator6/1 -> Data Type Conversion6/1
  Relational Operator5/1 -> Data Type Conversion5/1
  Relational Operator4/1 -> Data Type Conversion4/1
  Repeating Sequence8/1 -> Relational Operator8/1
  Repeating Sequence11/1 -> Relational Operator7/1
  Relational Operator9/1 -> Data Type Conversion9/1
  Relational Operator8/1 -> Data Type Conversion8/1
  Relational Operator7/1 -> Data Type Conversion7/1
  Data Type Conversion9/1 -> Gain4/1
  Data Type Conversion8/1 -> Gain3/1
  Data Type Conversion7/1 -> Gain2/1
  Repeating Sequence10/1 -> Relational Operator9/1
  Data Type Conversion4/1 -> Sum/1
  Data Type Conversion5/1 -> Sum/2
  Data Type Conversion6/1 -> Sum/3
  Data Type Conversion/1 -> Sum/4
  Data Type Conversion1/1 -> Sum/5
  Gain/1 -> Sum/6
  Gain1/1 -> Sum/7
  Gain2/1 -> Sum/8
  Gain3/1 -> Sum/9
  Gain4/1 -> Sum/10
  Sum/1 -> Scope4/1, LOOKUP TABLE/1(In1)

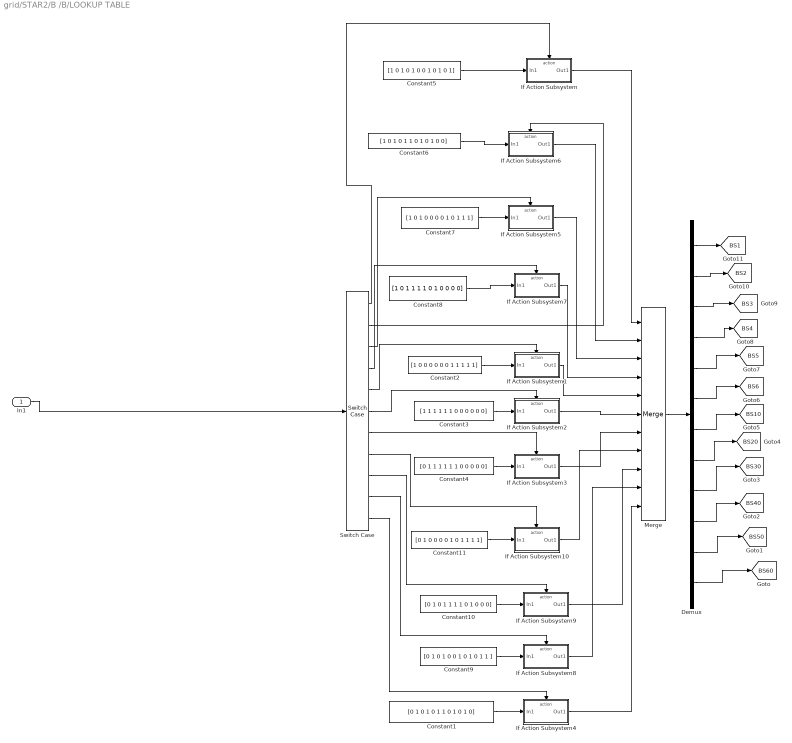
== system grid/STAR2/B /B/LOOKUP TABLE ==
  In1 : Inport
  Constant1 : Constant  Value=[0 1 0 1 0 1 1 0 1 0 1 0]
  Constant10 : Constant  Value=[0 1 0 1 1 1 1 0 1 0 0 0]
  Constant11 : Constant  Value=[0 1 0 0 0 0 1 0 1 1 1 1]
  Constant2 : Constant  Value=[1 0 0 0 0 0 0 1 1 1 1 1]
  Constant3 : Constant  Value=[1 1 1 1 1 1 0 0 0 0 0 0]
  Constant4 : Constant  Value=[0 1 1 1 1 1 1 0 0 0 0 0]
  Constant5 : Constant  Value=[1 0 1 0 1 0 0 1 0 1 0 1]
  Constant6 : Constant  Value=[1 0 1 0 1 1 0 1 0 1 0 0]
  Constant7 : Constant  Value=[1 0 1 0 0 0 0 1 0 1 1 1]
  Constant8 : Constant  Value=[1 0 1 1 1 1 0 1 0 0 0 0]
  Constant9 : Constant  Value=[0 1 0 1 0 0 1 0 1 0 1 1 ]
  Demux : Demux  Outputs=12
  If Action Subsystem : Subsystem  TreatAsAtomicUnit=on
  If Action Subsystem1 : Subsystem  TreatAsAtomicUnit=on
  If Action Subsystem10 : Subsystem  TreatAsAtomicUnit=on
  If Action Subsystem2 : Subsystem  TreatAsAtomicUnit=on
  If Action Subsystem3 : Subsystem  TreatAsAtomicUnit=on
  If Action Subsystem4 : Subsystem  TreatAsAtomicUnit=on
  If Action Subsystem5 : Subsystem  TreatAsAtomicUnit=on
  If Action Subsystem6 : Subsystem  TreatAsAtomicUnit=on
  If Action Subsystem7 : Subsystem  TreatAsAtomicUnit=on
  If Action Subsystem8 : Subsystem  TreatAsAtomicUnit=on
  If Action Subsystem9 : Subsystem  TreatAsAtomicUnit=on
  Merge : Merge  Inputs=11
  Switch Case : SwitchCase  CaseConditions={-5 -4 -3 -2 -1 0 1 2 3 4 5}  ShowDefaultCase=off
  tag scope: BS10=global, BS1=global, BS20=global, BS2=global, BS30=global, BS3=global, BS40=global, BS4=global, BS50=global, BS5=global, BS60=global, BS6=global
  wires:
  Demux/12 -> [BS60]
  Demux/9 -> [BS30]
  Demux/10 -> [BS40]
  Demux/11 -> [BS50]
  Demux/8 -> [BS20]
  Demux/7 -> [BS10]
  Demux/5 -> [BS5]
  Demux/6 -> [BS6]
  Demux/4 -> [BS4]
  Demux/3 -> [BS3]
  Demux/2 -> [BS2]
  Demux/1 -> [BS1]
  In1/1 -> Switch Case/1
  Constant5/1 -> If Action Subsystem/1(In1)
  Constant1/1 -> If Action Subsystem4/1(In1)
  If Action Subsystem8/1(Out1) -> Merge/10
  If Action Subsystem9/1(Out1) -> Merge/9
  If Action Subsystem10/1(Out1) -> Merge/8
  Constant8/1 -> If Action Subsystem7/1(In1)
  Constant7/1 -> If Action Subsystem5/1(In1)
  Constant6/1 -> If Action Subsystem6/1(In1)
  Switch Case/1 -> If Action Subsystem/Action
  Switch Case/2 -> If Action Subsystem6/Action
  Switch Case/3 -> If Action Subsystem5/Action
  Switch Case/4 -> If Action Subsystem7/Action
  Switch Case/5 -> If Action Subsystem1/Action
  Switch Case/7 -> If Action Subsystem3/Action
  Switch Case/8 -> If Action Subsystem10/Action
  Switch Case/9 -> If Action Subsystem9/Action
  Switch Case/10 -> If Action Subsystem8/Action
  If Action Subsystem4/1(Out1) -> Merge/11
  Switch Case/11 -> If Action Subsystem4/Action
  Constant11/1 -> If Action Subsystem10/1(In1)
  Constant10/1 -> If Action Subsystem9/1(In1)
  Constant9/1 -> If Action Subsystem8/1(In1)
  If Action Subsystem3/1(Out1) -> Merge/7
  If Action Subsystem2/1(Out1) -> Merge/6
  If Action Subsystem1/1(Out1) -> Merge/5
  If Action Subsystem7/1(Out1) -> Merge/4
  If Action Subsystem5/1(Out1) -> Merge/3
  If Action Subsystem6/1(Out1) -> Merge/2
  Switch Case/6 -> If Action Subsystem2/Action
  Constant2/1 -> If Action Subsystem1/1(In1)
  Constant3/1 -> If Action Subsystem2/1(In1)
  Constant4/1 -> If Action Subsystem3/1(In1)
  If Action Subsystem/1(Out1) -> Merge/1
  Merge/1 -> Demux/1

== system grid/STAR2/B /B/Subsystem ==
  Fcn : Fcn  Expr=u/410.6
  Product : Product
  Scope1 : Scope
      settings: YMin=-8  YMax=8  SaveName=ScopeData2
  Scope5 : Scope
      settings: YMin=-8  YMax=8  SaveName=ScopeData5
  Sine Wave : Sin  Amplitude=5*m  Frequency=2*pi*50  Phase=2*2.0944  SampleTime=0
  Out1 : Outport
  wires:
  Product/1 -> Scope5/1
  Fcn/1 -> Product/1, Scope1/1
  [Vrms] -> Fcn/1
  Sine Wave/1 -> Out1/1, Product/2

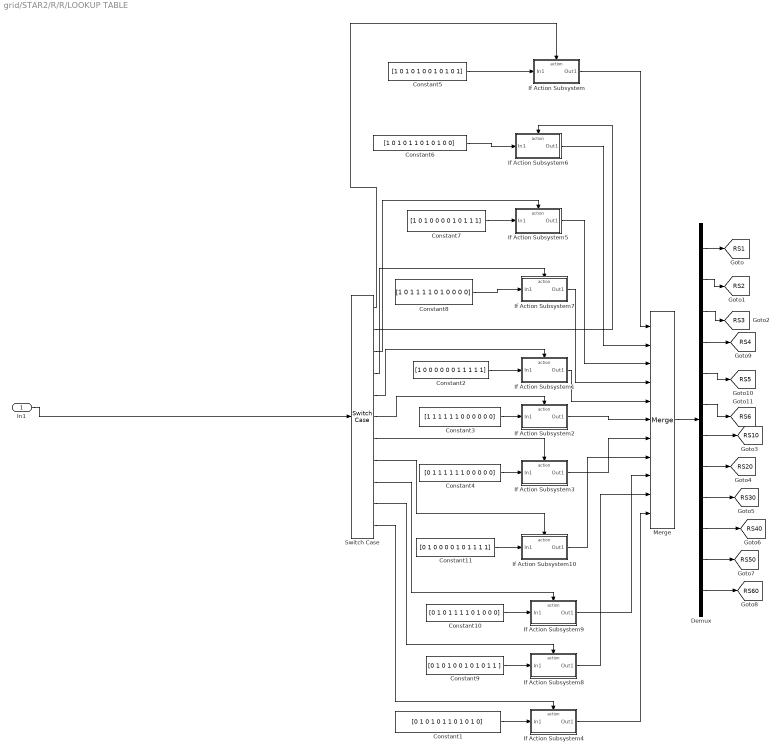
== system grid/STAR2/R/R/LOOKUP TABLE ==
  In1 : Inport
  Constant1 : Constant  Value=[0 1 0 1 0 1 1 0 1 0 1 0]
  Constant10 : Constant  Value=[0 1 0 1 1 1 1 0 1 0 0 0]
  Constant11 : Constant  Value=[0 1 0 0 0 0 1 0 1 1 1 1]
  Constant2 : Constant  Value=[1 0 0 0 0 0 0 1 1 1 1 1]
  Constant3 : Constant  Value=[1 1 1 1 1 1 0 0 0 0 0 0]
  Constant4 : Constant  Value=[0 1 1 1 1 1 1 0 0 0 0 0]
  Constant5 : Constant  Value=[1 0 1 0 1 0 0 1 0 1 0 1]
  Constant6 : Constant  Value=[1 0 1 0 1 1 0 1 0 1 0 0]
  Constant7 : Constant  Value=[1 0 1 0 0 0 0 1 0 1 1 1]
  Constant8 : Constant  Value=[1 0 1 1 1 1 0 1 0 0 0 0]
  Constant9 : Constant  Value=[0 1 0 1 0 0 1 0 1 0 1 1 ]
  Demux : Demux  Outputs=12
  If Action Subsystem : Subsystem  TreatAsAtomicUnit=on
  If Action Subsystem1 : Subsystem  TreatAsAtomicUnit=on
  If Action Subsystem10 : Subsystem  TreatAsAtomicUnit=on
  If Action Subsystem2 : Subsystem  TreatAsAtomicUnit=on
  If Action Subsystem3 : Subsystem  TreatAsAtomicUnit=on
  If Action Subsystem4 : Subsystem  TreatAsAtomicUnit=on
  If Action Subsystem5 : Subsystem  TreatAsAtomicUnit=on
  If Action Subsystem6 : Subsystem  TreatAsAtomicUnit=on
  If Action Subsystem7 : Subsystem  TreatAsAtomicUnit=on
  If Action Subsystem8 : Subsystem  TreatAsAtomicUnit=on
  If Action Subsystem9 : Subsystem  TreatAsAtomicUnit=on
  Merge : Merge  Inputs=11
  Switch Case : SwitchCase  CaseConditions={-5 -4 -3 -2 -1 0 1 2 3 4 5}  ShowDefaultCase=off
  tag scope: RS10=global, RS1=global, RS20=global, RS2=global, RS30=global, RS3=global, RS40=global, RS4=global, RS50=global, RS5=global, RS60=global, RS6=global
  wires:
  In1/1 -> Switch Case/1
  Constant5/1 -> If Action Subsystem/1(In1)
  Constant1/1 -> If Action Subsystem4/1(In1)
  Demux/4 -> [RS4]
  Demux/5 -> [RS5]
  Demux/6 -> [RS6]
  Demux/12 -> [RS60]
  Demux/11 -> [RS50]
  Demux/10 -> [RS40]
  Demux/9 -> [RS30]
  Demux/8 -> [RS20]
  Demux/7 -> [RS10]
  Demux/1 -> [RS1]
  Demux/2 -> [RS2]
  Demux/3 -> [RS3]
  If Action Subsystem8/1(Out1) -> Merge/10
  If Action Subsystem9/1(Out1) -> Merge/9
  If Action Subsystem10/1(Out1) -> Merge/8
  Constant8/1 -> If Action Subsystem7/1(In1)
  Constant7/1 -> If Action Subsystem5/1(In1)
  Constant6/1 -> If Action Subsystem6/1(In1)
  Switch Case/1 -> If Action Subsystem/Action
  Switch Case/2 -> If Action Subsystem6/Action
  Switch Case/3 -> If Action Subsystem5/Action
  Switch Case/4 -> If Action Subsystem7/Action
  Switch Case/5 -> If Action Subsystem1/Action
  Switch Case/7 -> If Action Subsystem3/Action
  Switch Case/8 -> If Action Subsystem10/Action
  Switch Case/9 -> If Action Subsystem9/Action
  Switch Case/10 -> If Action Subsystem8/Action
  If Action Subsystem4/1(Out1) -> Merge/11
  Switch Case/11 -> If Action Subsystem4/Action
  Constant11/1 -> If Action Subsystem10/1(In1)
  Constant10/1 -> If Action Subsystem9/1(In1)
  Constant9/1 -> If Action Subsystem8/1(In1)
  If Action Subsystem3/1(Out1) -> Merge/7
  If Action Subsystem2/1(Out1) -> Merge/6
  If Action Subsystem1/1(Out1) -> Merge/5
  If Action Subsystem7/1(Out1) -> Merge/4
  If Action Subsystem5/1(Out1) -> Merge/3
  If Action Subsystem6/1(Out1) -> Merge/2
  Switch Case/6 -> If Action Subsystem2/Action
  Constant2/1 -> If Action Subsystem1/1(In1)
  Constant3/1 -> If Action Subsystem2/1(In1)
  Constant4/1 -> If Action Subsystem3/1(In1)
  If Action Subsystem/1(Out1) -> Merge/1
  Merge/1 -> Demux/1

== system grid/STAR2/R/R/Subsystem ==
  Fcn : Fcn  Expr=u/410
  Product : Product
  Scope1 : Scope
      settings: YMin=-8  YMax=8  SaveName=ScopeData2
  Scope2 : Scope
      settings: YMin=-8  YMax=8  SaveName=ScopeData9
  Scope5 : Scope
      settings: YMin=-8  YMax=8  SaveName=ScopeData5
  Sine Wave : Sin  Amplitude=5*m  Frequency=2*pi*50  SampleTime=0
  Out1 : Outport
  wires:
  Product/1 -> Scope5/1
  Fcn/1 -> Product/1, Scope1/1
  [Vrms] -> Fcn/1, Scope2/1
  Sine Wave/1 -> Out1/1, Product/2

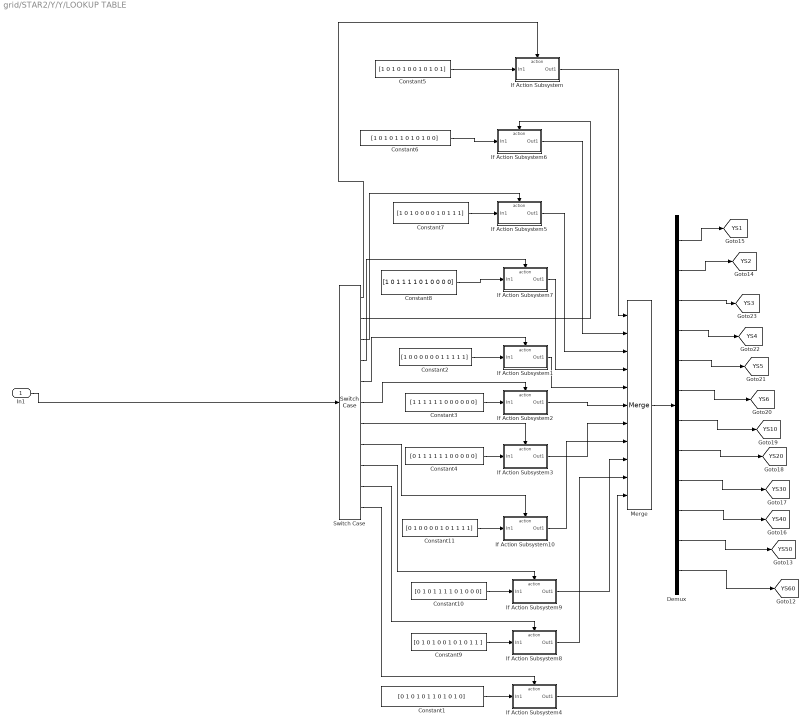
== system grid/STAR2/Y/Y/LOOKUP TABLE ==
  In1 : Inport
  Constant1 : Constant  Value=[0 1 0 1 0 1 1 0 1 0 1 0]
  Constant10 : Constant  Value=[0 1 0 1 1 1 1 0 1 0 0 0]
  Constant11 : Constant  Value=[0 1 0 0 0 0 1 0 1 1 1 1]
  Constant2 : Constant  Value=[1 0 0 0 0 0 0 1 1 1 1 1]
  Constant3 : Constant  Value=[1 1 1 1 1 1 0 0 0 0 0 0]
  Constant4 : Constant  Value=[0 1 1 1 1 1 1 0 0 0 0 0]
  Constant5 : Constant  Value=[1 0 1 0 1 0 0 1 0 1 0 1]
  Constant6 : Constant  Value=[1 0 1 0 1 1 0 1 0 1 0 0]
  Constant7 : Constant  Value=[1 0 1 0 0 0 0 1 0 1 1 1]
  Constant8 : Constant  Value=[1 0 1 1 1 1 0 1 0 0 0 0]
  Constant9 : Constant  Value=[0 1 0 1 0 0 1 0 1 0 1 1 ]
  Demux : Demux  Outputs=12
  If Action Subsystem : Subsystem  TreatAsAtomicUnit=on
  If Action Subsystem1 : Subsystem  TreatAsAtomicUnit=on
  If Action Subsystem10 : Subsystem  TreatAsAtomicUnit=on
  If Action Subsystem2 : Subsystem  TreatAsAtomicUnit=on
  If Action Subsystem3 : Subsystem  TreatAsAtomicUnit=on
  If Action Subsystem4 : Subsystem  TreatAsAtomicUnit=on
  If Action Subsystem5 : Subsystem  TreatAsAtomicUnit=on
  If Action Subsystem6 : Subsystem  TreatAsAtomicUnit=on
  If Action Subsystem7 : Subsystem  TreatAsAtomicUnit=on
  If Action Subsystem8 : Subsystem  TreatAsAtomicUnit=on
  If Action Subsystem9 : Subsystem  TreatAsAtomicUnit=on
  Merge : Merge  Inputs=11
  Switch Case : SwitchCase  CaseConditions={-5 -4 -3 -2 -1 0 1 2 3 4 5}  ShowDefaultCase=off
  tag scope: YS10=global, YS1=global, YS20=global, YS2=global, YS30=global, YS3=global, YS40=global, YS4=global, YS50=global, YS5=global, YS60=global, YS6=global
  wires:
  Demux/12 -> [YS60]
  Demux/11 -> [YS50]
  Demux/10 -> [YS40]
  Demux/9 -> [YS30]
  Demux/8 -> [YS20]
  Demux/7 -> [YS10]
  Demux/6 -> [YS6]
  Demux/5 -> [YS5]
  Demux/4 -> [YS4]
  Demux/2 -> [YS2]
  Demux/3 -> [YS3]
  Demux/1 -> [YS1]
  Merge/1 -> Demux/1
  If Action Subsystem/1(Out1) -> Merge/1
  Constant4/1 -> If Action Subsystem3/1(In1)
  Constant3/1 -> If Action Subsystem2/1(In1)
  Constant2/1 -> If Action Subsystem1/1(In1)
  Switch Case/6 -> If Action Subsystem2/Action
  If Action Subsystem6/1(Out1) -> Merge/2
  If Action Subsystem5/1(Out1) -> Merge/3
  If Action Subsystem7/1(Out1) -> Merge/4
  If Action Subsystem1/1(Out1) -> Merge/5
  If Action Subsystem2/1(Out1) -> Merge/6
  If Action Subsystem3/1(Out1) -> Merge/7
  Constant9/1 -> If Action Subsystem8/1(In1)
  Constant10/1 -> If Action Subsystem9/1(In1)
  Constant11/1 -> If Action Subsystem10/1(In1)
  Switch Case/11 -> If Action Subsystem4/Action
  If Action Subsystem4/1(Out1) -> Merge/11
  Switch Case/10 -> If Action Subsystem8/Action
  Switch Case/9 -> If Action Subsystem9/Action
  Switch Case/8 -> If Action Subsystem10/Action
  Switch Case/7 -> If Action Subsystem3/Action
  Switch Case/5 -> If Action Subsystem1/Action
  Switch Case/4 -> If Action Subsystem7/Action
  Switch Case/3 -> If Action Subsystem5/Action
  Switch Case/2 -> If Action Subsystem6/Action
  Switch Case/1 -> If Action Subsystem/Action
  Constant6/1 -> If Action Subsystem6/1(In1)
  Constant7/1 -> If Action Subsystem5/1(In1)
  Constant8/1 -> If Action Subsystem7/1(In1)
  If Action Subsystem10/1(Out1) -> Merge/8
  If Action Subsystem9/1(Out1) -> Merge/9
  If Action Subsystem8/1(Out1) -> Merge/10
  Constant1/1 -> If Action Subsystem4/1(In1)
  Constant5/1 -> If Action Subsystem/1(In1)
  In1/1 -> Switch Case/1

== system grid/STAR2/Y/Y/Subsystem ==
  Fcn : Fcn  Expr=u/410.6
  Product : Product
  Scope1 : Scope
      settings: YMin=-8  YMax=8  SaveName=ScopeData2
  Scope5 : Scope
      settings: YMin=-8  YMax=8  SaveName=ScopeData5
  Sine Wave : Sin  Amplitude=5*m  Frequency=2*pi*50  Phase=2.0944  SampleTime=0
  Out1 : Outport
  wires:
  Product/1 -> Scope5/1
  Fcn/1 -> Product/1, Scope1/1
  [Vrms] -> Fcn/1
  Sine Wave/1 -> Out1/1, Product/2

== system grid/STAR2/B /B/LOOKUP TABLE/If Action Subsystem ==
  In1 : Inport
  Action Port : ActionPort  ActionType=case
  Out1 : Outport
  wires:
  In1/1 -> Out1/1

== system grid/STAR2/B /B/LOOKUP TABLE/If Action Subsystem1 ==
  In1 : Inport
  Action Port : ActionPort  ActionType=case
  Out1 : Outport
  wires:
  In1/1 -> Out1/1

== system grid/STAR2/B /B/LOOKUP TABLE/If Action Subsystem10 ==
  In1 : Inport
  Action Port : ActionPort  ActionType=case
  Out1 : Outport
  wires:
  In1/1 -> Out1/1

== system grid/STAR2/B /B/LOOKUP TABLE/If Action Subsystem2 ==
  In1 : Inport
  Action Port : ActionPort  ActionType=case
  Out1 : Outport
  wires:
  In1/1 -> Out1/1

== system grid/STAR2/B /B/LOOKUP TABLE/If Action Subsystem3 ==
  In1 : Inport
  Action Port : ActionPort  ActionType=case
  Out1 : Outport
  wires:
  In1/1 -> Out1/1

== system grid/STAR2/B /B/LOOKUP TABLE/If Action Subsystem4 ==
  In1 : Inport
  Action Port : ActionPort  ActionType=case
  Out1 : Outport
  wires:
  In1/1 -> Out1/1

== system grid/STAR2/B /B/LOOKUP TABLE/If Action Subsystem5 ==
  In1 : Inport
  Action Port : ActionPort  ActionType=case
  Out1 : Outport
  wires:
  In1/1 -> Out1/1

== system grid/STAR2/B /B/LOOKUP TABLE/If Action Subsystem6 ==
  In1 : Inport
  Action Port : ActionPort  ActionType=case
  Out1 : Outport
  wires:
  In1/1 -> Out1/1

== system grid/STAR2/B /B/LOOKUP TABLE/If Action Subsystem7 ==
  In1 : Inport
  Action Port : ActionPort  ActionType=case
  Out1 : Outport
  wires:
  In1/1 -> Out1/1

== system grid/STAR2/B /B/LOOKUP TABLE/If Action Subsystem8 ==
  In1 : Inport
  Action Port : ActionPort  ActionType=case
  Out1 : Outport
  wires:
  In1/1 -> Out1/1

== system grid/STAR2/B /B/LOOKUP TABLE/If Action Subsystem9 ==
  In1 : Inport
  Action Port : ActionPort  ActionType=case
  Out1 : Outport
  wires:
  In1/1 -> Out1/1
